simulink model "c2812pwmtest"  (Simulink 6.0)
settings: Solver=FixedStepDiscrete  StartTime=0.0  StopTime=inf  RelTol=1e-3
libraries: c2800dspchiplib x1, c2000tgtpreflib x1
settings Model: Creator=zgalijas  LastModifiedBy=zgalijas  ProdHWDeviceType=TI C2000
settings DataIOCC: SaveOutput=off  SaveTime=off  SignalLoggingName=logsOut
settings OptimizationCC: InlineInvariantSignals=off
settings DebuggingCC: CheckExecutionContextPreStartOutputMsg=on  CheckExecutionContextRuntimeOutputMsg=on  SolverPrmCheckMsg=none
settings HardwareCC: ProdBitPerChar=16  ProdBitPerInt=16  ProdIntDivRoundTo=Zero  ProdEndianess=LittleEndian  ProdWordSize=16  ProdHWDeviceType=TI C2000  TargetHWDeviceType=32-bit Generic
settings ModelReferenceCC: UpdateModelReferenceTargets=IfOutOfDate
settings RTWCC: SystemTargetFile=ti_c2000_grt.tlc  TemplateMakefile=ti_c2000_grt.tmf  ProcessScript=ti_c2000_grt_make_rtw_hook
settings STFCustomTargetCC: TargetFcnLib=ansi_tfl_tmw.mat  GenFloatMathFcnCalls=ANSI_C  ModelReferenceCompliant=off  SystemTargetFile=ti_c2000_grt.tlc  ActivateCallback=ti_c2000_callback('ActivateCallback',hSrc,hDlg);  ForcedBaseTarget=off
settings GRTTargetCC: ModelReferenceCompliant=off  MatFileLogging=off
settings SFSimCC: SFSimApplyToAllLibs=on  SFSimBuildMode=Incremental

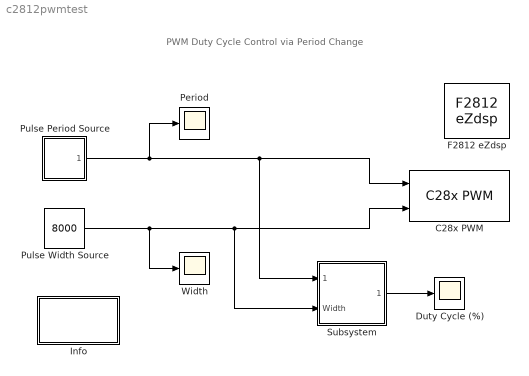
== system c2812pwmtest ==
  note: PWM Duty Cycle Control via Period Change
  " Info" : Subsystem  PropExecContextAcrossSSBoundary=on
      mask Display: disp('Info')
  C28x PWM : c2800dspchiplib/C28x PWM  useModule=A  timerSource=Input port  timerPeriod=64000  waveformType=Asymmetric  unit1Status=on  unit1Source=Input port  unit1Value=2000  unit2Status=off  unit2Source=Input port  unit2Value=2000  unit3Status=off  unit3Source=Input port  unit3Value=2000  unit1_1Logic=Active high  unit1_2Logic=Active low  unit2_1Logic=Active high  unit2_2Logic=Active low  unit3_1Logic=Active high  unit3_2Logic=Active low  enableDeadband1=off  enableDeadband2=off  enableDeadband3=off  deadbandPrescaler=1  deadbandPeriod=1  adcstartEvent=None
  Duty Cycle (%) : Scope
      settings: YMin=0  YMax=100  SaveName=ScopeData2
  F2812 eZdsp : c2000tgtpreflib/F2812 eZdsp  Tag=C2000 TARGET PREFERENCES BLOCK
  Period : Scope
      settings: YMin=8000  YMax=40000
  Pulse Period Source : Subsystem  PropExecContextAcrossSSBoundary=on
  Pulse Width Source : Constant  Value=8000  OutDataTypeMode=uint16  ConRadixGroup=Best Precision: Vector-wise  OutScaling=2^-10
  Subsystem : Subsystem  PropExecContextAcrossSSBoundary=on
  Width : Scope
      settings: YMin=0  YMax=16000
  wires:
  Pulse Width Source/1 -> Width/1, Subsystem/2(Width), C28x PWM/2
  Pulse Period Source/1(Period) -> Period/1, Subsystem/1(Period), C28x PWM/1
  Subsystem/1(Duty Cycle) -> Duty Cycle (%)/1

== system c2812pwmtest/ Info ==
  note: Demo Description:
  note: Setup:
  note: The code generation portion of this demo requires the following hardware:
      |
      | Spectrum Digital eZdsp F2812
      | Oscilloscope and probes
      |
      | Connect the output of PWM1 on the eZdsp F2812 to the analog input of the oscilloscope.
  note: This example demonstrates the use of the c2812 PWM block in generating the pulse
      | waveform.
      |
      | "Pulse Period Source" controls the period of the pulse waveform generated by the PWM1
      | and PWM2 of the eZdsp. The period is changing between 16000 and 32000 clock cycles.
      |
      | "Pulse Width Source" controls the width of the pulse waveform generated by the PWM1
      | and PWM2 of the eZdsp. The width is fixed to 8000 clock cycles.
      |
      | The duty cycle of the generated pulse waveform is determined by the relative ratio of the
      | pulse width and the pulse period. In this example, the duty cycle toggles between 50%
      | and 75% every 1.6 s. This effect can be observed on the oscilloscope.

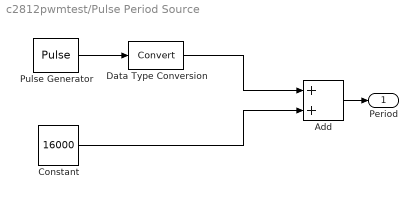
== system c2812pwmtest/Pulse Period Source ==
  Add : Sum  OutDataTypeMode=uint16  OutScaling=2^-10
  Constant : Constant  Value=16000  OutDataTypeMode=uint16  ConRadixGroup=Best Precision: Vector-wise  OutScaling=2^-10
  Data Type Conversion : DataTypeConversion  OutDataTypeMode=uint16  SaturateOnIntegerOverflow=on  RndMeth=Zero
  Pulse Generator : DiscretePulseGenerator  Amplitude=16000  Period=4000  PulseWidth=2000  SampleTime=64/80000
  Period : Outport
  wires:
  Pulse Generator/1 -> Data Type Conversion/1
  Data Type Conversion/1 -> Add/1
  Constant/1 -> Add/2
  Add/1 -> Period/1

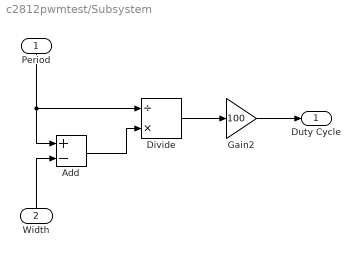
== system c2812pwmtest/Subsystem ==
  Period : Inport  Orientation=down  LatchInput=off
  Width : Inport  Orientation=up  Port=2  LatchInput=off
  Add : Sum  Inputs=+-  OutScaling=2^-10
  Divide : Product  Inputs=/*  OutDataTypeMode=single  OutScaling=2^-10
  Gain2 : Gain  Gain=100  ParameterScaling=2^-15  OutScaling=2^-10  SaturateOnIntegerOverflow=on
  Duty Cycle : Outport
  wires:
  Period/1 -> Divide/1, Add/1
  Divide/1 -> Gain2/1
  Gain2/1 -> Duty Cycle/1
  Add/1 -> Divide/2
  Width/1 -> Add/2
